simulink library "casper_library_scopes"  (Simulink 7.4)
settings: Solver=ode45  SolverMode=SingleTasking  StartTime=0.0  StopTime=10.0  RelTol=1e-3
libraries: xbsIndex_r4 x369, xps_library x28, casper_library_misc x12, casper_library_scopes x4, simulink x1
(part 1 of 4)
settings Model: Creator=mdexter  LastModifiedBy=griffin

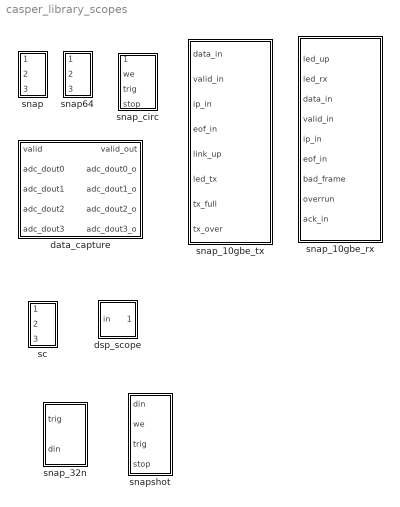
== system casper_library_scopes ==
  data_capture : Subsystem  mask(data_capture){stream_name=adc_dout, nsimult_streams=4}
      mask prompts: stream_name "Stream Name"; nsimult_streams "Number Of Simultaneous Streams"
      mask help:
      | This block is useful for capturing parallel data streams
      | simultaneously and sending the data in structures for analysis
      | using MATLAB.  It is intended as a partial replacement for the
      | Simulink scope block when used with the functions in data_capture_tools.
      |
      | The block does not alter the data at all and costs no hardware
      | because it is purely a simulation block.  The block's Simulink
      | outputs are exactly the same as its inputs with no delay.
      mask init:
      | data_capture_init(gcb, ...
      |     'stream_name', stream_name, ...
      |     'nsimult_streams', nsimult_streams);
  dsp_scope : Subsystem  mask(dsp_scope){n_inputs=32, slice_width=8, bin_pt=7, arith_type=1}
      mask prompts: n_inputs "Number of inputs"; slice_width "Width of each input"; bin_pt "Output Binary Point"; arith_type "Output Arithmetic Type (0=Unsigned, 1 = Signed)"
      mask help:
      | This block provides a convenient interface to plotting waveforms
      | of blocks with serial data output in parallel.  The core example
      | is of the ADC, which outputs 8 samples / clock.  This scope (simulation only)
      | samples sufficently fast (based on the number of parallel inputs)
      | to serialize the output for view in a standard simulink scope.
      |
      | The input must be concatenated parallel data streams, and
      | each data binary point must be 0.  The easiest way to do this is
      | to push  all the inputs through a "cram" block from the
      | GAVRT blockset.
      | easy
      mask init:
      | dsp_scope_init(gcb, ...
      |     'n_inputs', n_inputs, ...
      |     'slice_width', slice_width, ...
      |     'bin_pt', bin_pt, ...
      |     'arith_type', arith_type);
  sc : Subsystem  mask(sc){nsamples=11, offset=0}
      mask prompts: nsamples "No. of samples(2^?)"; offset "Parallel Bus Offset"
      mask help:
      | The 'sc' block is a modified version of the 'snap' block in
      | the same library.  The modification intends to move the software
      | register which has partial control over the 'we' line to the
      | bram as an external port so that multiple brams can use the same
      | gated write enable, i.e. they can share the software register
      | that enables writing to the bram.  This will simplify synchronous writing
      | to multiple brams.
      |
      | The 'sc' core is used in the 'snap_32n' block to mask the
      | 32-bit word limitation of the bram.
      mask init:
      | set_param([gcb, '/bram'], 'addr_width', num2str(nsamples));
      mask Help: eval('xlWeb(''http://casper.berkeley.edu/wiki/Snap'')')
  snap : Subsystem  mask(snap){nsamples=11}
      mask prompts: nsamples "No. of samples(2^?)"
      mask help:
      | The <i>snap</i> block provides a packaged solution to capturing data from
      | the FPGA fabric and making it accessible from the CPU.  The block comes in
      | 2 flavors: <i>snap</i> (which captures to a 32 bit wide Shared BRAM), and
      | <i>snap64</i> (which captures to 2x32 bit wide Shared BRAMs to effect a
      | 64 bit capture).
      mask init:
      | set_param([gcb, '/bram'], 'addr_width', num2str(nsamples));
      mask Help: eval('xlWeb(''http://casper.berkeley.edu/wiki/Snap'')')
  snap64 : Subsystem  mask(snap64){nsamples=11}
      mask prompts: nsamples "No. of samples(2^?)"
      mask help:
      | The <i>snap</i> block provides a packaged solution to capturing data from
      | the FPGA fabric and making it accessible from the CPU.  The block comes in
      | 2 flavors: <i>snap</i> (which captures to a 32 bit wide Shared BRAM), and
      | <i>snap64</i> (which captures to 2x32 bit wide Shared BRAMs to effect a
      | 64 bit capture).
      mask init:
      | set_param([gcb, '/bram_msb'], 'addr_width', num2str(nsamples));
      | set_param([gcb, '/bram_lsb'], 'addr_width', num2str(nsamples));
      mask Help: eval('xlWeb(''http://casper.berkeley.edu/wiki/Snap'')')
  snap_10gbe_rx : Subsystem  mask(snap_10gbe_rx){nsamples=11}
      mask prompts: nsamples "No. of samples(2^?)"
      mask help:
      | This snap block provides a packaged solution to capturing a 10GbE datastream from the FPGA fabric and making it accessible from the CPU.  The block captures data in 3 32-bit brams, two for the main data stream and one for out-of-band data (IP addresses, link status, buffer overflow warnings etc).
      |
      | There are two versions, one tailored for RX data streams and one tailored for TX data streams.
      mask init:
      | set_param([gcb, '/bram_oob'], 'addr_width', num2str(nsamples));
      | set_param([gcb, '/bram_msb'], 'addr_width', num2str(nsamples));
      | set_param([gcb, '/bram_lsb'], 'addr_width', num2str(nsamples));
  snap_10gbe_tx : Subsystem  mask(snap_10gbe_tx){nsamples=11}
      mask prompts: nsamples "No. of samples(2^?)"
      mask help:
      | This snap block provides a packaged solution to capturing a 10GbE datastream from the FPGA fabric and making it accessible from the CPU.  The block captures data in 3 32-bit brams, two for the main data stream and one for out-of-band data (IP addresses, link status, buffer overflow warnings etc).
      |
      | There are two versions, one tailored for RX data streams and one tailored for TX data streams.
      mask init:
      | set_param([gcb, '/bram_oob'], 'addr_width', num2str(nsamples));
      | set_param([gcb, '/bram_msb'], 'addr_width', num2str(nsamples));
      | set_param([gcb, '/bram_lsb'], 'addr_width', num2str(nsamples));
  snap_32n : Subsystem  mask(snap_32n){nsamples=11, width=4}
      mask prompts: nsamples "Number of Samples (2^"; width "Input Bus Width (32x"
      mask help:
      | Like the snap64 block, this block contains multiple sub-cores
      | that each have a separate bram.  The purpose is to be able to
      | extend the functionality of the 'snap' and 'sc' blocks to beyond
      | the 32-bit word limitation of a single bram by synchronously
      | writing different parts of a larger bus to separate BRAMs.  UNLIKE
      | the snap64 block, the bus width on the 'snap_32n' block is
      | parameterizable to any multiple of 32.
      mask init:
      | snap_32n_init(gcb, ...
      |     'nsamples', nsamples, ...
      |     'width', width);
  snap_circ : Subsystem  mask(snap_circ){nsamples=10}
      mask prompts: nsamples "Number of Samples (2^?)"
      mask help:
      | Backwards compatible with the normal snap block, but with the following upgrades:
      |  1) Ability to offset the trigger. Optionally delay the fabric trigger by a user-specified number of valids.
      |  2) 'Addr' register's MSb now indicates 'busy capturing'.
      |  3) Ability to capture continuously until a stop pulse is received. Data is captured into BRAM continuously, with old data being overwritten until a stop command is received. Then stop capturing when memory is filled. This enables you to get some data before and some data after the stop pulse. Use the 'tr_en_cnt' register to determine where you are in your vector.
      mask init:
      | set_param([gcb, '/bram'], 'addr_width', num2str(nsamples));
  snapshot : Subsystem  mask(snapshot){storage=bram, dram_dimm=1, dram_clock=200, nsamples=10, data_width=32, offset=on, circap=on, value=off, use_dsp48=on}
      mask prompts: storage "Storage medium"; dram_dimm "DRAM dimm"; dram_clock "DRAM clock rate"; nsamples "Number of Samples (2^?)"; data_width "Data width"; offset "Start delay support"; circap "Circular capture support"; value "Extra value capture support"; use_dsp48 "Use DSP48s to implement counters"
      mask help:
      | Standard snap block, but with the following optional extras;
      |  1) Optionally delay the fabric trigger by a user-specified number of valids.
      |  2) Capture continuously after a trigger until a stop pulse is received. Data is captured into BRAM continuously, with old data being overwritten until a stop command is received. Then stop capturing when memory is filled. This enables you to get some data before and some data after the stop pulse. Use the 'tr_en_cnt' register to determine where you are in your vector. 'Addr' register's MSb now indicates 'busy capturing'.
      |  3) Optionally capture a value on an input port to a register at the same time as the first data sample.
      |  4) Implement counters using DSP48Es to save resources.
      mask init:
      | snapshot_init(gcb, ...
      |     'storage', storage, ...
      |     'dram_dimm', dram_dimm, ...
      |     'dram_clock', dram_clock, ...
      |     'nsamples', nsamples, ...
      |     'data_width', data_width, ...
      |     'offset', offset, ...
      |     'circap', circap, ...
      |     'value', value, ...
      |     'use_dsp48', use_dsp48);
      mask StyleString: popup(bram|dram),popup(1|2|3|4),popup(200|250|266|300|333),edit,popup(8|16|32|64|128),checkbox,checkbox,checkbox,checkbox
      mask CallbackString: snapshot_callback();||||||||

== system casper_library_scopes/data_capture ==
  valid : Inport  OutDataType=sfix(16)  OutScaling=2^0
  adc_dout0 : Inport  Port=2  OutDataType=sfix(16)  OutScaling=2^0
  adc_dout1 : Inport  Port=3  OutDataType=sfix(16)  OutScaling=2^0
  adc_dout2 : Inport  Port=4  OutDataType=sfix(16)  OutScaling=2^0
  adc_dout3 : Inport  Port=5  OutDataType=sfix(16)  OutScaling=2^0
  ToWorkspace_adc_dout0 : ToWorkspace  VariableName=adc_dout0  SampleTime=-1  SaveFormat=Structure
  ToWorkspace_adc_dout1 : ToWorkspace  VariableName=adc_dout1  SampleTime=-1  SaveFormat=Structure
  ToWorkspace_adc_dout2 : ToWorkspace  VariableName=adc_dout2  SampleTime=-1  SaveFormat=Structure
  ToWorkspace_adc_dout3 : ToWorkspace  VariableName=adc_dout3  SampleTime=-1  SaveFormat=Structure
  ToWorkspace_valid : ToWorkspace  VariableName=adc_dout_valid  SampleTime=-1  SaveFormat=Structure
  valid_out : Outport  OutDataType=sfix(16)  OutScaling=2^0
  adc_dout0_o : Outport  Port=2  OutDataType=sfix(16)  OutScaling=2^0
  adc_dout1_o : Outport  Port=3  OutDataType=sfix(16)  OutScaling=2^0
  adc_dout2_o : Outport  Port=4  OutDataType=sfix(16)  OutScaling=2^0
  adc_dout3_o : Outport  Port=5  OutDataType=sfix(16)  OutScaling=2^0
  wires:
  adc_dout3/1 -> adc_dout3_o/1, ToWorkspace_adc_dout3/1
  adc_dout2/1 -> adc_dout2_o/1, ToWorkspace_adc_dout2/1
  adc_dout1/1 -> adc_dout1_o/1, ToWorkspace_adc_dout1/1
  adc_dout0/1 -> adc_dout0_o/1, ToWorkspace_adc_dout0/1
  valid/1 -> valid_out/1, ToWorkspace_valid/1

== system casper_library_scopes/dsp_scope ==
  in : Inport  OutDataType=sfix(16)  OutScaling=2^0
  sel : simulink/Sources/Counter Free-Running  SystemSampleTime=-1  NumBits=5  tsamp=0.03125
  switch : MultiPortSwitch  Inputs=32  zeroidx=on  OutDataType=sfix(16)  OutScaling=2^0
  uncram : Subsystem  AncestorBlock=gavrt_library/uncram  mask(uncram){num_slice=32, slice_width=8, bin_pt=7, arith_type=1}
      mask prompts: num_slice "Number of slices"; slice_width "Slice Width"; bin_pt "Output Binary Point"; arith_type "Output Arithmetic Type (0=Unsigned, 1=Signed)"
      mask help: Takes a concatenated input and slices it up into even pieces and reinterprets them as signed fixed point numbers with a given binary point.
      mask init:
      | uncram_init(gcb, ...
      |     'num_slice', num_slice, ...
      |     'slice_width', slice_width, ...
      |     'bin_pt', bin_pt, ...
      |     'arith_type', arith_type);
      settings: AttributesFormatString=Fix_8_7
  out : Outport  OutDataType=sfix(16)  OutScaling=2^0
  wires:
  in/1 -> uncram/1(In)
  switch/1 -> out/1
  sel/1 -> switch/1
  uncram/1(Out1) -> switch/2
  uncram/2(Out2) -> switch/3
  uncram/3(Out3) -> switch/4
  uncram/4(Out4) -> switch/5
  uncram/5(Out5) -> switch/6
  uncram/6(Out6) -> switch/7
  uncram/7(Out7) -> switch/8
  uncram/8(Out8) -> switch/9
  uncram/9(Out9) -> switch/10
  uncram/10(Out10) -> switch/11
  uncram/11(Out11) -> switch/12
  uncram/12(Out12) -> switch/13
  uncram/13(Out13) -> switch/14
  uncram/14(Out14) -> switch/15
  uncram/15(Out15) -> switch/16
  uncram/16(Out16) -> switch/17
  uncram/17(Out17) -> switch/18
  uncram/18(Out18) -> switch/19
  uncram/19(Out19) -> switch/20
  uncram/20(Out20) -> switch/21
  uncram/21(Out21) -> switch/22
  uncram/22(Out22) -> switch/23
  uncram/23(Out23) -> switch/24
  uncram/24(Out24) -> switch/25
  uncram/25(Out25) -> switch/26
  uncram/26(Out26) -> switch/27
  uncram/27(Out27) -> switch/28
  uncram/28(Out28) -> switch/29
  uncram/29(Out29) -> switch/30
  uncram/30(Out30) -> switch/31
  uncram/31(Out31) -> switch/32
  uncram/32(Out32) -> switch/33

== system casper_library_scopes/sc ==
  din : Inport  OutDataType=sfix(16)  OutScaling=2^0
  trig : Inport  Port=2  OutDataType=sfix(16)  OutScaling=2^0
  read_freeze : Inport  Port=3  OutDataType=sfix(16)  OutScaling=2^0
  Constant : xbsIndex_r4/Constant  arith_type=Unsigned  const=2^nsamples  n_bits=32  bin_pt=0  explicit_period=on  period=1  equ=P=C  opselect=C  inp2=PCIN>>17  opr=+  inp1=P  carry=CIN  dbl_ovrd=off  block_type=constant
  Counter : xbsIndex_r4/Counter  cnt_type=Count Limited  cnt_to=Inf  operation=Up  start_count=0  cnt_by_val=1  arith_type=Unsigned  n_bits=nsamples+1  bin_pt=0  load_pin=off  rst=on  en=off  explicit_period=on  period=1  dbl_ovrd=off  use_behavioral_HDL=off  implementation=Fabric  use_rpm=off  block_type=counter
  Inverter : xbsIndex_r4/Inverter  en=off  latency=0  dbl_ovrd=off  block_type=inv
  Logical : xbsIndex_r4/Logical  logical_function=AND  inputs=2  en=off  latency=0  precision=Full  arith_type=Unsigned  n_bits=16  bin_pt=0  align_bp=on  dbl_ovrd=off  block_type=logical
  Reinterpret : xbsIndex_r4/Reinterpret  force_arith_type=on  arith_type=Unsigned  force_bin_pt=on  bin_pt=0  block_type=reinterpret
      settings: infoedit="Changes signal type without altering the binary representation.   You can changed the signal between signed and unsigned, and relocate the binary point.<P><P>Hardware notes: In hardware this block costs nothing.<P><P>Example:  Suppose the input is 6 bits wide, signed, with 2 fractional bits, and the output is forced to unsigned with 0 fractional bits.  Then an input of -2.0 (1110.00 in binary 2's complement) becomes an output of 56 (111000 in binary)."  block_version=10.1.1
  Relational : xbsIndex_r4/Relational  mode=a<b  en=off  latency=1  dbl_ovrd=off  block_type=relational
      settings: block_version=10.1.3
  Slice : xbsIndex_r4/Slice  nbits=1  boolean_output=on  mode=Lower Bit Location + Width  bit1=0  base1=MSB of Input  bit0=0  base0=LSB of Input  dbl_ovrd=off  block_type=slice
      settings: infoedit="Extracts a given range of bits from each input sample and presents it at the output.  The output type is ordinarily unsigned with binary point at zero, but can be Boolean when the slice is one bit wide.<P><P>Hardware notes: In hardware this block costs nothing."  block_version=10.1.3
  bram : xps_library/Shared BRAM  Tag=xps:bram  SystemSampleTime=-1  arith_type=Unsigned  addr_width=11  data_width=32  data_bin_pt=0  init_vals=0  sample_rate=1
  data_sl : xbsIndex_r4/Slice  nbits=32  boolean_output=off  mode=Lower Bit Location + Width  bit1=0  base1=MSB of Input  bit0=offset  base0=LSB of Input  dbl_ovrd=off  block_type=slice
      settings: infoedit="Extracts a given range of bits from each input sample and presents it at the output.  The output type is ordinarily unsigned with binary point at zero, but can be Boolean when the slice is one bit wide.<P><P>Hardware notes: In hardware this block costs nothing."  block_version=10.1.3
  wires:
  data_sl/1 -> Reinterpret/1
  Constant/1 -> Relational/2
  Relational/1 -> bram/3
  read_freeze/1 -> Slice/1
  Slice/1 -> Inverter/1
  Logical/1 -> Counter/1
  Inverter/1 -> Logical/2
  trig/1 -> Logical/1
  Counter/1 -> Relational/1, bram/1
  Reinterpret/1 -> bram/2
  din/1 -> data_sl/1

== system casper_library_scopes/snap ==
  din : Inport  OutDataType=sfix(16)  OutScaling=2^0
  trig : Inport  Port=2  OutDataType=sfix(16)  OutScaling=2^0
  we : Inport  Port=3  OutDataType=sfix(16)  OutScaling=2^0
  Constant : xbsIndex_r4/Constant  arith_type=Boolean  const=1  n_bits=1  bin_pt=0  explicit_period=on  period=1  equ=P=C  opselect=C  inp2=PCIN>>17  opr=+  inp1=P  carry=CIN  dbl_ovrd=off  block_type=constant
      settings: block_version=10.1.1
  Constant1 : xbsIndex_r4/Constant  arith_type=Boolean  const=1  n_bits=1  bin_pt=0  explicit_period=on  period=1  equ=P=C  opselect=C  inp2=PCIN>>17  opr=+  inp1=P  carry=CIN  dbl_ovrd=off  block_type=constant
      settings: block_version=10.1.1
  Constant13 : Constant  OutDataType=sfix(16)  OutScaling=2^0
  Constant2 : xbsIndex_r4/Constant  arith_type=Boolean  const=1  n_bits=1  bin_pt=0  explicit_period=on  period=1  equ=P=C  opselect=C  inp2=PCIN>>17  opr=+  inp1=P  carry=CIN  dbl_ovrd=off  block_type=constant
      settings: block_version=10.1.1
  Inverter : xbsIndex_r4/Inverter  en=off  latency=0  dbl_ovrd=off  block_type=inv
      settings: xl_area=[0, 0, 0, 0, 0, 0, 0]  block_version=10.1.1
  Logical1 : xbsIndex_r4/Logical  logical_function=AND  inputs=2  en=off  latency=0  precision=Full  arith_type=Unsigned  n_bits=8  bin_pt=2  align_bp=on  dbl_ovrd=off  block_type=logical
      settings: xl_area=[0, 0, 0, 0, 0, 0, 0]  block_version=10.1.1
  Mux1 : xbsIndex_r4/Mux  inputs=2  en=off  latency=0  precision=Full  arith_type="Signed  (2's comp)"  n_bits=8  bin_pt=2  quantization=Truncate  overflow=Wrap  dbl_ovrd=off  block_type=mux
      settings: xl_area=[0, 0, 0, 0, 0, 0, 0]  block_version=10.1.1
  Mux2 : xbsIndex_r4/Mux  inputs=2  en=off  latency=0  precision=Full  arith_type="Signed  (2's comp)"  n_bits=8  bin_pt=2  quantization=Truncate  overflow=Wrap  dbl_ovrd=off  block_type=mux
      settings: xl_area=[0, 0, 0, 0, 0, 0, 0]  block_version=10.1.1
  Register : xbsIndex_r4/Register  init=0  rst=on  en=on  dbl_ovrd=off  block_type=register
      settings: xl_area=[0, 0, 0, 0, 0, 0, 0]  block_version=10.1.1
  Register1 : xbsIndex_r4/Register  init=0  rst=on  en=on  dbl_ovrd=off  block_type=register
      settings: xl_area=[0, 0, 0, 0, 0, 0, 0]  block_version=10.1.1
  Reinterpret : xbsIndex_r4/Reinterpret  force_arith_type=on  arith_type=Unsigned  force_bin_pt=on  bin_pt=0  block_type=reinterpret
      settings: infoedit="Changes signal type without altering the binary representation.   You can changed the signal between signed and unsigned, and relocate the binary point.<P><P>Hardware notes: In hardware this block costs nothing.<P><P>Example:  Suppose the input is 6 bits wide, signed, with 2 fractional bits, and the output is forced to unsigned with 0 fractional bits.  Then an input of -2.0 (1110.00 in binary 2's complement) becomes an output of 56 (111000 in binary)."  block_version=10.1.1
  addr : xps_library/software register  Tag=xps:sw_reg  SystemSampleTime=-1  io_dir=To Processor  arith_type=Unsigned  bitwidth=32  bin_pt=0  sample_period=1  gw_name=casper_library_Scopes_snap_addr_user_data_in
  bram : xps_library/Shared BRAM  Tag=xps:bram  SystemSampleTime=-1  arith_type=Unsigned  addr_width=11  data_width=32  data_bin_pt=0  init_vals=0  sample_rate=1
  ctrl : xps_library/software register  Tag=xps:sw_reg  SystemSampleTime=-1  io_dir=From Processor  arith_type=Unsigned  bitwidth=32  bin_pt=0  sample_period=1  gw_name=casper_library_Scopes_snap_ctrl_user_data_out
  enable : xbsIndex_r4/Slice  nbits=1  boolean_output=on  mode=Lower Bit Location + Width  bit1=0  base1=LSB of Input  bit0=0  base0=LSB of Input  dbl_ovrd=off  block_type=slice
      settings: infoedit="Extracts a given range of bits from each input sample and presents it at the output.  The output type is ordinarily unsigned with binary point at zero, but can be Boolean when the slice is one bit wide.<P><P>Hardware notes: In hardware this block costs nothing."  block_version=10.1.1
  freeze_cntr : casper_library_misc/freeze_cntr  SystemSampleTime=-1  CounterBits=nsamples
  posedge : casper_library_misc/posedge  Tag=Rising Edge Detector  SystemSampleTime=-1
  trig1 : xbsIndex_r4/Slice  nbits=1  boolean_output=on  mode=Lower Bit Location + Width  bit1=0  base1=LSB of Input  bit0=1  base0=LSB of Input  dbl_ovrd=off  block_type=slice
      settings: infoedit="Extracts a given range of bits from each input sample and presents it at the output.  The output type is ordinarily unsigned with binary point at zero, but can be Boolean when the slice is one bit wide.<P><P>Hardware notes: In hardware this block costs nothing."  block_version=10.1.1
  valid : xbsIndex_r4/Slice  nbits=1  boolean_output=on  mode=Lower Bit Location + Width  bit1=0  base1=LSB of Input  bit0=2  base0=LSB of Input  dbl_ovrd=off  block_type=slice
      settings: infoedit="Extracts a given range of bits from each input sample and presents it at the output.  The output type is ordinarily unsigned with binary point at zero, but can be Boolean when the slice is one bit wide.<P><P>Hardware notes: In hardware this block costs nothing."  block_version=10.1.1
  wires:
  Mux2/1 -> Logical1/1
  Inverter/1 -> Logical1/2
  Logical1/1 -> Register/2
  valid/1 -> Mux1/1
  trig1/1 -> Mux2/1
  Register1/1 -> addr/1
  Constant2/1 -> Mux1/3
  we/1 -> Mux1/2
  Mux1/1 -> freeze_cntr/1
  Constant1/1 -> Mux2/3
  Constant/1 -> Register/1
  posedge/1 -> Inverter/1, Register1/2, Register/3
  ctrl/1 -> trig1/1, valid/1, enable/1
  din/1 -> Reinterpret/1
  Reinterpret/1 -> bram/2
  Constant13/1 -> ctrl/1
  freeze_cntr/2 -> Register1/3, bram/3
  Register/1 -> freeze_cntr/2
  enable/1 -> posedge/1
  freeze_cntr/1 -> bram/1, Register1/1
  trig/1 -> Mux2/2

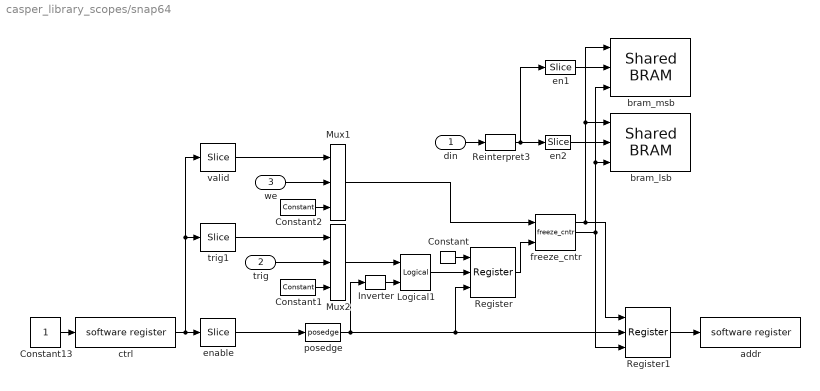
== system casper_library_scopes/snap64 ==
  din : Inport  OutDataType=sfix(16)  OutScaling=2^0
  trig : Inport  Port=2  OutDataType=sfix(16)  OutScaling=2^0
  we : Inport  Port=3  OutDataType=sfix(16)  OutScaling=2^0
  Constant : xbsIndex_r4/Constant  arith_type=Boolean  const=1  n_bits=1  bin_pt=0  explicit_period=on  period=1  equ=P=C  opselect=C  inp2=PCIN>>17  opr=+  inp1=P  carry=CIN  dbl_ovrd=off  block_type=constant
      settings: block_version=10.1.1
  Constant1 : xbsIndex_r4/Constant  arith_type=Boolean  const=1  n_bits=1  bin_pt=0  explicit_period=on  period=1  equ=P=C  opselect=C  inp2=PCIN>>17  opr=+  inp1=P  carry=CIN  dbl_ovrd=off  block_type=constant
      settings: block_version=10.1.1
  Constant13 : Constant  OutDataType=sfix(16)  OutScaling=2^0
  Constant2 : xbsIndex_r4/Constant  arith_type=Boolean  const=1  n_bits=1  bin_pt=0  explicit_period=on  period=1  equ=P=C  opselect=C  inp2=PCIN>>17  opr=+  inp1=P  carry=CIN  dbl_ovrd=off  block_type=constant
      settings: block_version=10.1.1
  Inverter : xbsIndex_r4/Inverter  en=off  latency=0  dbl_ovrd=off  block_type=inv
      settings: xl_area=[0, 0, 0, 0, 0, 0, 0]  block_version=10.1.1
  Logical1 : xbsIndex_r4/Logical  logical_function=AND  inputs=2  en=off  latency=0  precision=Full  arith_type=Unsigned  n_bits=8  bin_pt=2  align_bp=on  dbl_ovrd=off  block_type=logical
      settings: xl_area=[0, 0, 0, 0, 0, 0, 0]  block_version=10.1.1
  Mux1 : xbsIndex_r4/Mux  inputs=2  en=off  latency=0  precision=Full  arith_type="Signed  (2's comp)"  n_bits=8  bin_pt=2  quantization=Truncate  overflow=Wrap  dbl_ovrd=off  block_type=mux
      settings: xl_area=[0, 0, 0, 0, 0, 0, 0]  block_version=10.1.1
  Mux2 : xbsIndex_r4/Mux  inputs=2  en=off  latency=0  precision=Full  arith_type="Signed  (2's comp)"  n_bits=8  bin_pt=2  quantization=Truncate  overflow=Wrap  dbl_ovrd=off  block_type=mux
      settings: xl_area=[0, 0, 0, 0, 0, 0, 0]  block_version=10.1.1
  Register : xbsIndex_r4/Register  init=0  rst=on  en=on  dbl_ovrd=off  block_type=register
      settings: xl_area=[0, 0, 0, 0, 0, 0, 0]  block_version=10.1.1
  Register1 : xbsIndex_r4/Register  init=0  rst=on  en=on  dbl_ovrd=off  block_type=register
      settings: xl_area=[0, 0, 0, 0, 0, 0, 0]  block_version=10.1.1
  Reinterpret3 : xbsIndex_r4/Reinterpret  force_arith_type=on  arith_type=Unsigned  force_bin_pt=on  bin_pt=0  block_type=reinterpret
      settings: infoedit="Changes signal type without altering the binary representation.   You can changed the signal between signed and unsigned, and relocate the binary point.<P><P>Hardware notes: In hardware this block costs nothing.<P><P>Example:  Suppose the input is 6 bits wide, signed, with 2 fractional bits, and the output is forced to unsigned with 0 fractional bits.  Then an input of -2.0 (1110.00 in binary 2's complement) becomes an output of 56 (111000 in binary)."  block_version=10.1.1
  addr : xps_library/software register  Tag=xps:sw_reg  SystemSampleTime=-1  io_dir=To Processor  arith_type=Unsigned  bitwidth=32  bin_pt=0  sample_period=1  gw_name=casper_library_scopes_snap64_addr_user_data_in
  bram_lsb : xps_library/Shared BRAM  Tag=xps:bram  SystemSampleTime=-1  arith_type=Unsigned  addr_width=nsamples  data_width=32  data_bin_pt=0  init_vals=0  sample_rate=1
  bram_msb : xps_library/Shared BRAM  Tag=xps:bram  SystemSampleTime=-1  arith_type=Unsigned  addr_width=nsamples  data_width=32  data_bin_pt=0  init_vals=0  sample_rate=1
  ctrl : xps_library/software register  Tag=xps:sw_reg  SystemSampleTime=-1  io_dir=From Processor  arith_type=Unsigned  bitwidth=32  bin_pt=0  sample_period=1  gw_name=casper_library_scopes_snap64_ctrl_user_data_out
  en1 : xbsIndex_r4/Slice  nbits=32  boolean_output=off  mode=Lower Bit Location + Width  bit1=0  base1=LSB of Input  bit0=32  base0=LSB of Input  dbl_ovrd=off  block_type=slice
      settings: infoedit="Extracts a given range of bits from each input sample and presents it at the output.  The output type is ordinarily unsigned with binary point at zero, but can be Boolean when the slice is one bit wide.<P><P>Hardware notes: In hardware this block costs nothing."  block_version=10.1.1
  en2 : xbsIndex_r4/Slice  nbits=32  boolean_output=off  mode=Lower Bit Location + Width  bit1=0  base1=LSB of Input  bit0=0  base0=LSB of Input  dbl_ovrd=off  block_type=slice
      settings: infoedit="Extracts a given range of bits from each input sample and presents it at the output.  The output type is ordinarily unsigned with binary point at zero, but can be Boolean when the slice is one bit wide.<P><P>Hardware notes: In hardware this block costs nothing."  block_version=10.1.1
  enable : xbsIndex_r4/Slice  nbits=1  boolean_output=on  mode=Lower Bit Location + Width  bit1=0  base1=LSB of Input  bit0=0  base0=LSB of Input  dbl_ovrd=off  block_type=slice
      settings: infoedit="Extracts a given range of bits from each input sample and presents it at the output.  The output type is ordinarily unsigned with binary point at zero, but can be Boolean when the slice is one bit wide.<P><P>Hardware notes: In hardware this block costs nothing."  block_version=10.1.1
  freeze_cntr : casper_library_misc/freeze_cntr  SystemSampleTime=-1  CounterBits=nsamples
  posedge : casper_library_misc/posedge  Tag=Rising Edge Detector  SystemSampleTime=-1
  trig1 : xbsIndex_r4/Slice  nbits=1  boolean_output=on  mode=Lower Bit Location + Width  bit1=0  base1=LSB of Input  bit0=1  base0=LSB of Input  dbl_ovrd=off  block_type=slice
      settings: infoedit="Extracts a given range of bits from each input sample and presents it at the output.  The output type is ordinarily unsigned with binary point at zero, but can be Boolean when the slice is one bit wide.<P><P>Hardware notes: In hardware this block costs nothing."  block_version=10.1.1
  valid : xbsIndex_r4/Slice  nbits=1  boolean_output=on  mode=Lower Bit Location + Width  bit1=0  base1=LSB of Input  bit0=2  base0=LSB of Input  dbl_ovrd=off  block_type=slice
      settings: infoedit="Extracts a given range of bits from each input sample and presents it at the output.  The output type is ordinarily unsigned with binary point at zero, but can be Boolean when the slice is one bit wide.<P><P>Hardware notes: In hardware this block costs nothing."  block_version=10.1.1
  wires:
  freeze_cntr/1 -> bram_lsb/1, bram_msb/1, Register1/1
  Register/1 -> freeze_cntr/2
  Mux2/1 -> Logical1/1
  Inverter/1 -> Logical1/2
  Logical1/1 -> Register/2
  valid/1 -> Mux1/1
  trig1/1 -> Mux2/1
  Register1/1 -> addr/1
  Constant2/1 -> Mux1/3
  we/1 -> Mux1/2
  Mux1/1 -> freeze_cntr/1
  Constant1/1 -> Mux2/3
  Constant/1 -> Register/1
  posedge/1 -> Inverter/1, Register1/2, Register/3
  ctrl/1 -> trig1/1, valid/1, enable/1
  Constant13/1 -> ctrl/1
  freeze_cntr/2 -> bram_lsb/3, bram_msb/3, Register1/3
  enable/1 -> posedge/1
  trig/1 -> Mux2/2
  Reinterpret3/1 -> en1/1, en2/1
  din/1 -> Reinterpret3/1
  en1/1 -> bram_msb/2
  en2/1 -> bram_lsb/2

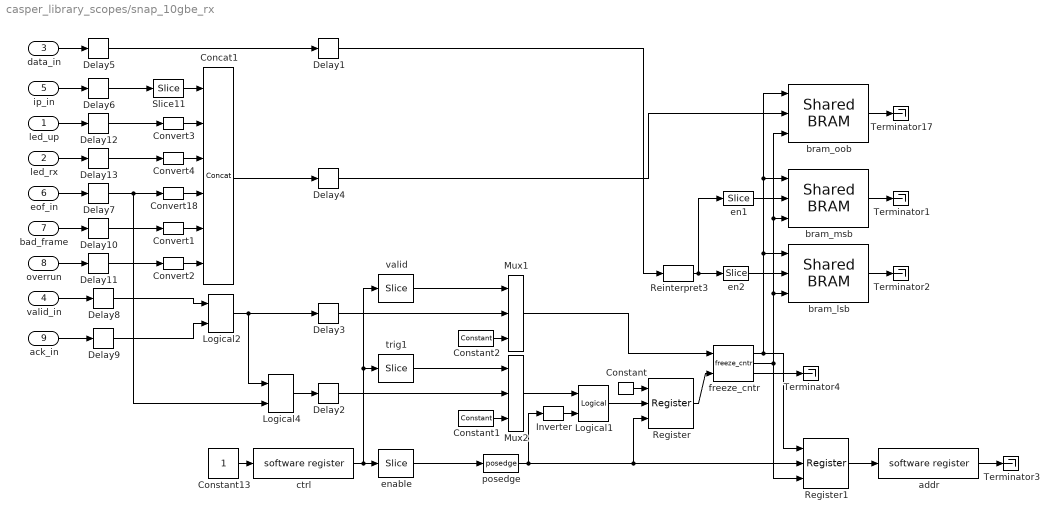
== system casper_library_scopes/snap_10gbe_rx ==
  led_up : Inport  OutDataType=sfix(16)  OutScaling=2^0
  led_rx : Inport  Port=2  OutDataType=sfix(16)  OutScaling=2^0
  data_in : Inport  Port=3  OutDataType=sfix(16)  OutScaling=2^0
  valid_in : Inport  Port=4  OutDataType=sfix(16)  OutScaling=2^0
  ip_in : Inport  Port=5  OutDataType=sfix(16)  OutScaling=2^0
  eof_in : Inport  Port=6  OutDataType=sfix(16)  OutScaling=2^0
  bad_frame : Inport  Port=7  OutDataType=sfix(16)  OutScaling=2^0
  overrun : Inport  Port=8  OutDataType=sfix(16)  OutScaling=2^0
  ack_in : Inport  Port=9  OutDataType=sfix(16)  OutScaling=2^0
  Concat1 : xbsIndex_r4/Concat  num_inputs=6  dbl_ovrd=off  block_type=concat
      settings: block_version=10.1.3
  Constant : xbsIndex_r4/Constant  arith_type=Boolean  const=1  n_bits=1  bin_pt=0  explicit_period=on  period=1  equ=P=C  opselect=C  inp2=PCIN>>17  opr=+  inp1=P  carry=CIN  dbl_ovrd=off  block_type=constant
  Constant1 : xbsIndex_r4/Constant  arith_type=Boolean  const=1  n_bits=1  bin_pt=0  explicit_period=on  period=1  equ=P=C  opselect=C  inp2=PCIN>>17  opr=+  inp1=P  carry=CIN  dbl_ovrd=off  block_type=constant
  Constant13 : Constant  OutDataType=sfix(16)  OutScaling=2^0
  Constant2 : xbsIndex_r4/Constant  arith_type=Boolean  const=1  n_bits=1  bin_pt=0  explicit_period=on  period=1  equ=P=C  opselect=C  inp2=PCIN>>17  opr=+  inp1=P  carry=CIN  dbl_ovrd=off  block_type=constant
  Convert{1..4,18} (5 alike) : xbsIndex_r4/Convert  arith_type=Unsigned  n_bits=1  bin_pt=0  quantization=Truncate  overflow=Wrap  latency=0  dbl_ovrd=off  pipeline=off  block_type=convert
      settings: xl_area=[0, 0, 0, 0, 0, 0, 0]  block_version=10.1.3
  Delay{1..13} (13 alike) : xbsIndex_r4/Delay  en=off  latency=2  dbl_ovrd=off  reg_retiming=on  block_type=delay
      settings: xl_area=[0, 0, 0, 0, 0, 0, 0]
  Inverter : xbsIndex_r4/Inverter  en=off  latency=0  dbl_ovrd=off  block_type=inv
      settings: xl_area=[0, 0, 0, 0, 0, 0, 0]
  Logical1 : xbsIndex_r4/Logical  logical_function=AND  inputs=2  en=off  latency=0  precision=Full  arith_type=Unsigned  n_bits=8  bin_pt=2  align_bp=on  dbl_ovrd=off  block_type=logical
      settings: xl_area=[0, 0, 0, 0, 0, 0, 0]
  Logical2 : xbsIndex_r4/Logical  logical_function=AND  inputs=2  en=off  latency=0  precision=Full  arith_type=Unsigned  n_bits=8  bin_pt=2  align_bp=on  dbl_ovrd=off  block_type=logical
      settings: xl_area=[0, 0, 0, 0, 0, 0, 0]
  Logical4 : xbsIndex_r4/Logical  logical_function=AND  inputs=2  en=off  latency=0  precision=Full  arith_type=Unsigned  n_bits=8  bin_pt=2  align_bp=on  dbl_ovrd=off  block_type=logical
      settings: xl_area=[0, 0, 0, 0, 0, 0, 0]
  Mux1 : xbsIndex_r4/Mux  inputs=2  en=off  latency=0  precision=Full  arith_type="Signed  (2's comp)"  n_bits=8  bin_pt=2  quantization=Truncate  overflow=Wrap  dbl_ovrd=off  block_type=mux
      settings: xl_area=[0, 0, 0, 0, 0, 0, 0]
  Mux2 : xbsIndex_r4/Mux  inputs=2  en=off  latency=0  precision=Full  arith_type="Signed  (2's comp)"  n_bits=8  bin_pt=2  quantization=Truncate  overflow=Wrap  dbl_ovrd=off  block_type=mux
      settings: xl_area=[0, 0, 0, 0, 0, 0, 0]
  Register : xbsIndex_r4/Register  init=0  rst=on  en=on  dbl_ovrd=off  block_type=register
      settings: xl_area=[0, 0, 0, 0, 0, 0, 0]
  Register1 : xbsIndex_r4/Register  init=0  rst=on  en=on  dbl_ovrd=off  block_type=register
      settings: xl_area=[0, 0, 0, 0, 0, 0, 0]
  Reinterpret3 : xbsIndex_r4/Reinterpret  force_arith_type=on  arith_type=Unsigned  force_bin_pt=on  bin_pt=0  block_type=reinterpret
      settings: infoedit="Changes signal type without altering the binary representation.   You can changed the signal between signed and unsigned, and relocate the binary point.<P><P>Hardware notes: In hardware this block costs nothing.<P><P>Example:  Suppose the input is 6 bits wide, signed, with 2 fractional bits, and the output is forced to unsigned with 0 fractional bits.  Then an input of -2.0 (1110.00 in binary 2's complement) becomes an output of 56 (111000 in binary)."  block_version=10.1.3
  Slice11 : xbsIndex_r4/Slice  nbits=32-5  boolean_output=off  mode=Lower Bit Location + Width  bit1=0  base1=MSB of Input  bit0=0  base0=LSB of Input  dbl_ovrd=off  block_type=slice
      settings: infoedit="Extracts a given range of bits from each input sample and presents it at the output.  The output type is ordinarily unsigned with binary point at zero, but can be Boolean when the slice is one bit wide.<P><P>Hardware notes: In hardware this block costs nothing."  block_version=10.1.3
  Terminator{1..4,17} (5 alike) : Terminator
  addr : xps_library/software register  Tag=xps:sw_reg  SystemSampleTime=-1  io_dir=To Processor  arith_type=Unsigned  bitwidth=32  bin_pt=0  sample_period=1  gw_name=casper_library_scopes_snap_10gbe_rx_addr_user_data_in
      link override convert: arith_type=Unsigned  n_bits=32  bin_pt=0
  bram_lsb : xps_library/Shared BRAM  Tag=xps:bram  SystemSampleTime=-1  arith_type=Unsigned  addr_width=11  data_width=32  data_bin_pt=0  init_vals=0  sample_rate=1
      link override b_2x_8a_r310b_snap_gbe_rx0_bram_lsb_data_out: arith_type=Unsigned
      link override convert_din: arith_type=Unsigned
      link override mem/sim_data_in: arith_type=Unsigned
      link override r_10gbe_demo_snap_gbe0_rx_bram_lsb_data_out: arith_type=Unsigned
      link override r_10gbe_test_snap_gbe0_rx_bram_lsb_data_out: arith_type=Unsigned
      link override r_2x_8a_r310b_snap_gbe_rx0_bram_lsb_data_out: arith_type=Unsigned
      link override r_2x_8a_r311a_snap_gbe_rx0_bram_lsb_data_out: arith_type=Unsigned
      link override r_2x_8a_r311b_snap_gbe_rx0_bram_lsb_data_out: arith_type=Unsigned
  bram_msb : xps_library/Shared BRAM  Tag=xps:bram  SystemSampleTime=-1  arith_type=Unsigned  addr_width=11  data_width=32  data_bin_pt=0  init_vals=0  sample_rate=1
      link override b_2x_8a_r310b_snap_gbe_rx0_bram_msb_data_out: arith_type=Unsigned
      link override convert_din: arith_type=Unsigned
      link override mem/sim_data_in: arith_type=Unsigned
      link override r_10gbe_demo_snap_gbe0_rx_bram_msb_data_out: arith_type=Unsigned
      link override r_10gbe_test_snap_gbe0_rx_bram_msb_data_out: arith_type=Unsigned
      link override r_2x_8a_r310b_snap_gbe_rx0_bram_msb_data_out: arith_type=Unsigned
      link override r_2x_8a_r311a_snap_gbe_rx0_bram_msb_data_out: arith_type=Unsigned
      link override r_2x_8a_r311b_snap_gbe_rx0_bram_msb_data_out: arith_type=Unsigned
  bram_oob : xps_library/Shared BRAM  Tag=xps:bram  SystemSampleTime=-1  arith_type=Unsigned  addr_width=11  data_width=32  data_bin_pt=0  init_vals=0  sample_rate=1
      link override b_2x_8a_r310b_snap_gbe_rx0_bram_oob_data_out: arith_type=Unsigned
      link override convert_din: arith_type=Unsigned
      link override mem/sim_data_in: arith_type=Unsigned
      link override r_10gbe_demo_snap_gbe0_rx_bram_oob_data_out: arith_type=Unsigned
      link override r_10gbe_test_snap_gbe0_rx_bram_oob_data_out: arith_type=Unsigned
      link override r_2x_8a_r310b_snap_gbe_rx0_bram_oob_data_out: arith_type=Unsigned
      link override r_2x_8a_r311a_snap_gbe_rx0_bram_oob_data_out: arith_type=Unsigned
      link override r_2x_8a_r311b_snap_gbe_rx0_bram_oob_data_out: arith_type=Unsigned
  ctrl : xps_library/software register  Tag=xps:sw_reg  SystemSampleTime=-1  io_dir=From Processor  arith_type=Unsigned  bitwidth=32  bin_pt=0  sample_period=1  gw_name=casper_library_scopes_snap_10gbe_rx_ctrl_user_data_out
      link override b_2x_8a_r310b_snap_gbe_rx0_ctrl_user_data_out: arith_type=Unsigned  n_bits=32  bin_pt=0  period=1
      link override r_10gbe_demo_snap_gbe0_rx_ctrl_user_data_out: arith_type=Unsigned  n_bits=32  bin_pt=0  period=1
      link override r_10gbe_test_snap_gbe0_rx_ctrl_user_data_out: arith_type=Unsigned  n_bits=32  bin_pt=0  period=1
      link override r_2x_8a_r310b_snap_gbe_rx0_ctrl_user_data_out: arith_type=Unsigned  n_bits=32  bin_pt=0  period=1
      link override r_2x_8a_r311a_snap_gbe_rx0_ctrl_user_data_out: arith_type=Unsigned  n_bits=32  bin_pt=0  period=1
      link override r_2x_8a_r311b_snap_gbe_rx0_ctrl_user_data_out: arith_type=Unsigned  n_bits=32  bin_pt=0  period=1
  en1 : xbsIndex_r4/Slice  nbits=32  boolean_output=off  mode=Lower Bit Location + Width  bit1=0  base1=LSB of Input  bit0=32  base0=LSB of Input  dbl_ovrd=off  block_type=slice
      settings: infoedit="Extracts a given range of bits from each input sample and presents it at the output.  The output type is ordinarily unsigned with binary point at zero, but can be Boolean when the slice is one bit wide.<P><P>Hardware notes: In hardware this block costs nothing."  block_version=10.1.3
  en2 : xbsIndex_r4/Slice  nbits=32  boolean_output=off  mode=Lower Bit Location + Width  bit1=0  base1=LSB of Input  bit0=0  base0=LSB of Input  dbl_ovrd=off  block_type=slice
      settings: infoedit="Extracts a given range of bits from each input sample and presents it at the output.  The output type is ordinarily unsigned with binary point at zero, but can be Boolean when the slice is one bit wide.<P><P>Hardware notes: In hardware this block costs nothing."  block_version=10.1.3
  enable : xbsIndex_r4/Slice  nbits=1  boolean_output=on  mode=Lower Bit Location + Width  bit1=0  base1=LSB of Input  bit0=0  base0=LSB of Input  dbl_ovrd=off  block_type=slice
      settings: infoedit="Extracts a given range of bits from each input sample and presents it at the output.  The output type is ordinarily unsigned with binary point at zero, but can be Boolean when the slice is one bit wide.<P><P>Hardware notes: In hardware this block costs nothing."  block_version=10.1.3
  freeze_cntr : casper_library_misc/freeze_cntr  SystemSampleTime=-1  CounterBits=nsamples
  posedge : casper_library_misc/posedge  Tag=Rising Edge Detector  SystemSampleTime=-1
  trig1 : xbsIndex_r4/Slice  nbits=1  boolean_output=on  mode=Lower Bit Location + Width  bit1=0  base1=LSB of Input  bit0=1  base0=LSB of Input  dbl_ovrd=off  block_type=slice
      settings: infoedit="Extracts a given range of bits from each input sample and presents it at the output.  The output type is ordinarily unsigned with binary point at zero, but can be Boolean when the slice is one bit wide.<P><P>Hardware notes: In hardware this block costs nothing."  block_version=10.1.3
  valid : xbsIndex_r4/Slice  nbits=1  boolean_output=on  mode=Lower Bit Location + Width  bit1=0  base1=LSB of Input  bit0=2  base0=LSB of Input  dbl_ovrd=off  block_type=slice
      settings: infoedit="Extracts a given range of bits from each input sample and presents it at the output.  The output type is ordinarily unsigned with binary point at zero, but can be Boolean when the slice is one bit wide.<P><P>Hardware notes: In hardware this block costs nothing."  block_version=10.1.3
  wires:
  addr/1 -> Terminator3/1
  freeze_cntr/3 -> Terminator4/1
  bram_lsb/1 -> Terminator2/1
  bram_msb/1 -> Terminator1/1
  bram_oob/1 -> Terminator17/1
  Convert2/1 -> Concat1/6
  Convert1/1 -> Concat1/5
  Convert18/1 -> Concat1/4
  Convert4/1 -> Concat1/3
  Convert3/1 -> Concat1/2
  Slice11/1 -> Concat1/1
  Delay13/1 -> Convert4/1
  led_rx/1 -> Delay13/1
  Delay12/1 -> Convert3/1
  led_up/1 -> Delay12/1
  Delay11/1 -> Convert2/1
  overrun/1 -> Delay11/1
  Delay10/1 -> Convert1/1
  bad_frame/1 -> Delay10/1
  Delay9/1 -> Logical2/2
  Delay8/1 -> Logical2/1
  Delay7/1 -> Logical4/2, Convert18/1
  Delay6/1 -> Slice11/1
  Delay5/1 -> Delay1/1
  Delay3/1 -> Mux1/2
  Delay2/1 -> Mux2/2
  Logical2/1 -> Logical4/1, Delay3/1
  ack_in/1 -> Delay9/1
  eof_in/1 -> Delay7/1
  valid_in/1 -> Delay8/1
  Logical4/1 -> Delay2/1
  Delay4/1 -> bram_oob/2
  Delay1/1 -> Reinterpret3/1
  ip_in/1 -> Delay6/1
  data_in/1 -> Delay5/1
  Concat1/1 -> Delay4/1
  en2/1 -> bram_lsb/2
  en1/1 -> bram_msb/2
  Reinterpret3/1 -> en2/1, en1/1
  enable/1 -> posedge/1
  freeze_cntr/2 -> Register1/3, bram_oob/3, bram_msb/3, bram_lsb/3
  Constant13/1 -> ctrl/1
  ctrl/1 -> enable/1, valid/1, trig1/1
  posedge/1 -> Register/3, Register1/2, Inverter/1
  Constant/1 -> Register/1
  Constant1/1 -> Mux2/3
  Mux1/1 -> freeze_cntr/1
  Constant2/1 -> Mux1/3
  Register1/1 -> addr/1
  trig1/1 -> Mux2/1
  valid/1 -> Mux1/1
  Logical1/1 -> Register/2
  Inverter/1 -> Logical1/2
  Mux2/1 -> Logical1/1
  Register/1 -> freeze_cntr/2
  freeze_cntr/1 -> Register1/1, bram_oob/1, bram_msb/1, bram_lsb/1
